simulink model "Wahadlo_model_lin"  (R2015a)
settings: Solver=ode45  SolverMode=SingleTasking  StartTime=0.0  StopTime=20  FixedStep=0.001  RelTol=1e-3  AbsTol=1e-6
values from neighbouring files (symbols this model uses):
  l0 = [0 0 0 0]    [model_prep_lqr.m]    (also in model_prep_swingup.m)
undefined symbols (not defined in the file or in its folder): a, b, g, l, M, m, s, w
settings Model: ExtModeTrigDuration=12000  ExtModeTrigLevel=0.400000  Creator=jims  LastModifiedBy=omicronns
settings DataIOCC: ExternalInput=[]  InitialState=[]  LimitDataPoints=off  MaxDataPoints=5000  SignalLoggingSaveFormat=ModelDataLogs  SaveOutput=off  SaveTime=off  SignalLoggingName=sigsOut
settings OptimizationCC: BooleanDataType=off  ExpressionDepthLimit=2147483647  InitFltsAndDblsToZero=on
settings DebuggingCC: SaveWithParameterizedLinksMsg=none  UnderspecifiedInitializationDetection=Classic  MergeDetectMultiDrivingBlocksExec=none  SignalResolutionControl=TryResolveAllWithWarning  MultiTaskDSMMsg=warning  MultiTaskCondExecSysMsg=none  IntegerOverflowMsg=none  FcnCallInpInsideContextMsg=UseLocalSettings  StateNameClashWarn=warning  IntegerSaturationMsg=none
settings HardwareCC: ProdBitPerLong=64  ProdBitPerPointer=64  ProdIntDivRoundTo=Zero  ProdEndianess=LittleEndian  ProdWordSize=64  ProdHWDeviceType=Intel->x86-64  TargetBitPerLong=64  TargetBitPerPointer=64  TargetIntDivRoundTo=Zero  TargetEndianess=LittleEndian  TargetWordSize=64  TargetHWDeviceType=Intel->x86-64
settings RTWCC: SystemTargetFile=rtwin.tlc  TemplateMakefile=RTDAC_win.tmf  Description=Real-Time Windows Target
settings RTWinTargetCC: TargetFcnLib=ansi_tfl_tmw.mat  TargetPreCompLibLocation=C:\Program Files\MATLAB\MATLAB Production Server\R2015a\toolbox\sldrt\lib\win64  ModelReferenceCompliant=off  CompOptLevelCompliant=off

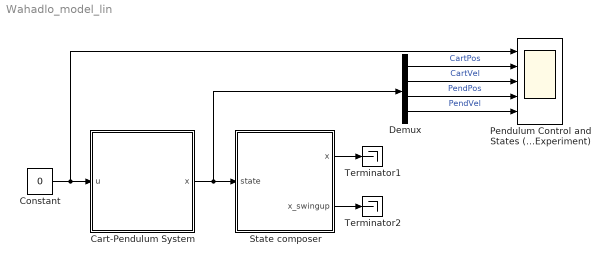
== system Wahadlo_model_lin ==
  Cart-Pendulum System : Subsystem
  Constant : Constant  Value=0
  Demux : Demux
  Pendulum Control and States (Experiment) : Scope  NumInputPorts=5
      settings: TimeRange=10  YMin=-0.2~-0.01~-0.04~0~-10  YMax=0.1~0.004999999999999999~0.02~6~10  SaveName=P1_Data  MaxDataPoints=50000
  State composer : Subsystem
  Terminator1 : Terminator
  Terminator2 : Terminator
  wires:
  Demux/4 -> Pendulum Control and States (Experiment)/5  "PendVel"
  Demux/3 -> Pendulum Control and States (Experiment)/4  "PendPos"
  Demux/2 -> Pendulum Control and States (Experiment)/3  "CartVel"
  Demux/1 -> Pendulum Control and States (Experiment)/2  "CartPos"
  Constant/1 -> Cart-Pendulum System/1(u), Pendulum Control and States (Experiment)/1
  Cart-Pendulum System/1(x) -> Demux/1, State composer/1(state)
  State composer/1(x) -> Terminator1/1
  State composer/2(x_swingup) -> Terminator2/1

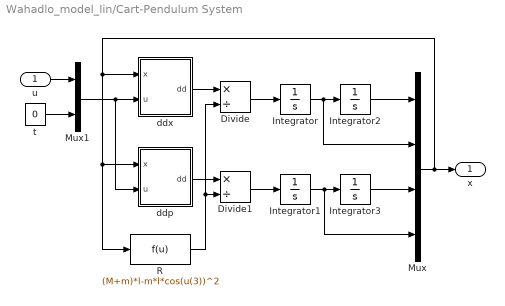
== system Wahadlo_model_lin/Cart-Pendulum System ==
  u : Inport
  Divide : Product  Inputs=*/
  Divide1 : Product  Inputs=*/
  Integrator : Integrator  InitialCondition=l0(2)
  Integrator1 : Integrator  InitialCondition=l0(4)
  Integrator2 : Integrator  InitialCondition=l0(1)
  Integrator3 : Integrator  InitialCondition=l0(3)
  Mux : Mux
  Mux1 : Mux  Inputs=2
  R : Fcn  Expr=(M+m)*l-m*l*cos(u(3))^2
  ddp : Subsystem
  ddx : Subsystem
  t : Constant  Value=0
  x : Outport
  wires:
  Integrator/1 -> Mux/2, Integrator2/1
  Integrator1/1 -> Mux/4, Integrator3/1
  Integrator2/1 -> Mux/1
  Integrator3/1 -> Mux/3
  Mux/1 -> R/1, ddp/1(x), ddx/1(x), x/1
  ddx/1(dd) -> Divide/1
  ddp/1(dd) -> Divide1/1
  Divide/1 -> Integrator/1
  Divide1/1 -> Integrator1/1
  R/1 -> Divide/2, Divide1/2
  Mux1/1 -> ddp/2(u), ddx/2(u)
  t/1 -> Mux1/2
  u/1 -> Mux1/1

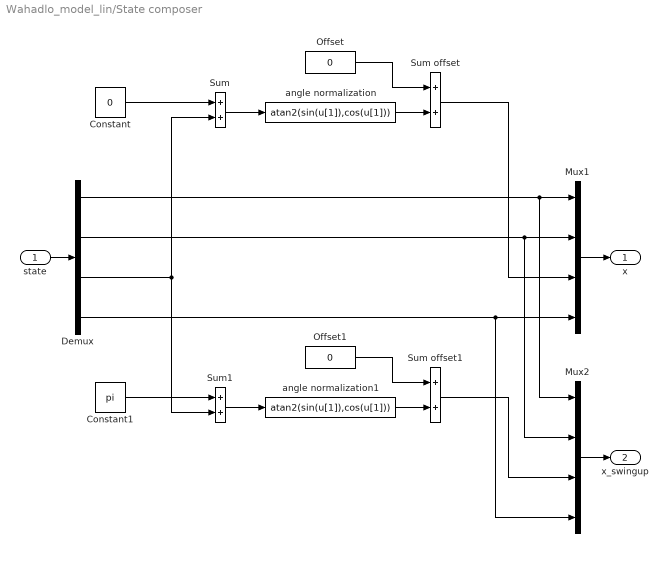
== system Wahadlo_model_lin/State composer ==
  state : Inport
  Constant : Constant  Value=0
  Constant1 : Constant  Value=pi
  Demux : Demux
  Mux1 : Mux
  Mux2 : Mux
  Offset : Constant  Value=0
  Offset1 : Constant  Value=0
  Sum : Sum  SaturateOnIntegerOverflow=on  InputSameDT=on  OutDataTypeStr=Inherit: Same as first input
  Sum offset : Sum  SaturateOnIntegerOverflow=on  InputSameDT=on  OutDataTypeStr=Inherit: Same as first input
  Sum offset1 : Sum  SaturateOnIntegerOverflow=on  InputSameDT=on  OutDataTypeStr=Inherit: Same as first input
  Sum1 : Sum  SaturateOnIntegerOverflow=on  InputSameDT=on  OutDataTypeStr=Inherit: Same as first input
  angle normalization : Fcn  Expr=atan2(sin(u[1]),cos(u[1]))
  angle normalization1 : Fcn  Expr=atan2(sin(u[1]),cos(u[1]))
  x : Outport  InitialOutput=0
  x_swingup : Outport  Port=2  InitialOutput=0
  wires:
  angle normalization/1 -> Sum offset/2
  Offset/1 -> Sum offset/1
  Sum/1 -> angle normalization/1
  Constant/1 -> Sum/1
  Mux1/1 -> x/1
  angle normalization1/1 -> Sum offset1/2
  Offset1/1 -> Sum offset1/1
  Sum1/1 -> angle normalization1/1
  Constant1/1 -> Sum1/1
  Mux2/1 -> x_swingup/1
  Sum offset/1 -> Mux1/3
  state/1 -> Demux/1
  Demux/3 -> Sum1/2, Sum/2
  Demux/2 -> Mux1/2, Mux2/2
  Demux/1 -> Mux1/1, Mux2/1
  Demux/4 -> Mux2/4, Mux1/4
  Sum offset1/1 -> Mux2/3

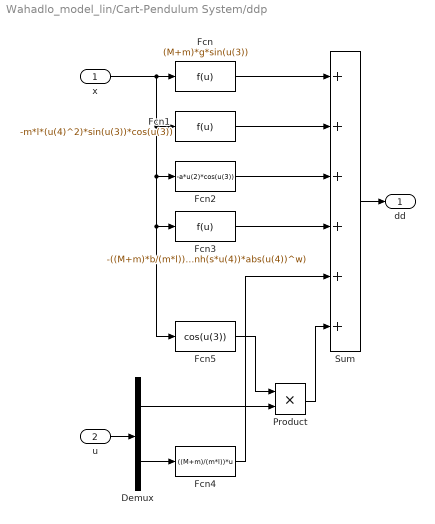
== system Wahadlo_model_lin/Cart-Pendulum System/ddp ==
  x : Inport
  u : Inport  Port=2
  Demux : Demux  Outputs=2
  Fcn : Fcn  Expr=(M+m)*g*sin(u(3))
  Fcn1 : Fcn  Expr=-m*l*(u(4)^2)*sin(u(3))*cos(u(3))
  Fcn2 : Fcn  Expr=-a*u(2)*cos(u(3))
  Fcn3 : Fcn  Expr=-((M+m)*b/(m*l))*(tanh(s*u(4))*abs(u(4))^w)
  Fcn4 : Fcn  Expr=((M+m)/(m*l))*u
  Fcn5 : Fcn  Expr=cos(u(3))
  Product : Product
  Sum : Sum  Inputs=++++++
  dd : Outport
  wires:
  u/1 -> Demux/1
  Fcn5/1 -> Product/1
  Fcn/1 -> Sum/1
  Fcn1/1 -> Sum/2
  Fcn2/1 -> Sum/3
  Fcn3/1 -> Sum/4
  x/1 -> Fcn3/1, Fcn5/1, Fcn2/1, Fcn1/1, Fcn/1
  Product/1 -> Sum/6
  Sum/1 -> dd/1
  Demux/2 -> Fcn4/1
  Demux/1 -> Product/2
  Fcn4/1 -> Sum/5

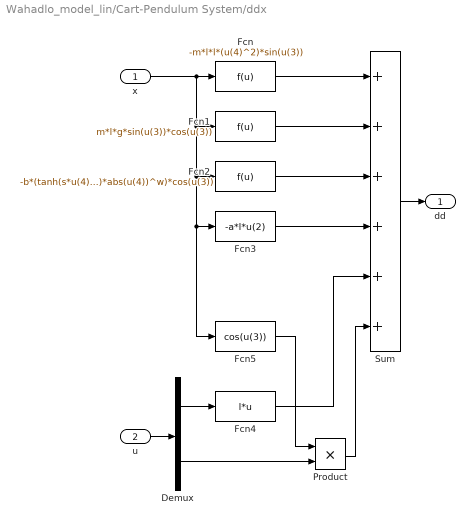
== system Wahadlo_model_lin/Cart-Pendulum System/ddx ==
  x : Inport
  u : Inport  Port=2
  Demux : Demux  Outputs=2
  Fcn : Fcn  Expr=-m*l*l*(u(4)^2)*sin(u(3))
  Fcn1 : Fcn  Expr=m*l*g*sin(u(3))*cos(u(3))
  Fcn2 : Fcn  Expr=-b*(tanh(s*u(4))*abs(u(4))^w)*cos(u(3))
  Fcn3 : Fcn  Expr=-a*l*u(2)
  Fcn4 : Fcn  Expr=l*u
  Fcn5 : Fcn  Expr=cos(u(3))
  Product : Product
  Sum : Sum  Inputs=++++++
  dd : Outport
  wires:
  u/1 -> Demux/1
  Demux/1 -> Fcn4/1
  Fcn5/1 -> Product/1
  Demux/2 -> Product/2
  Fcn/1 -> Sum/1
  Fcn1/1 -> Sum/2
  Fcn2/1 -> Sum/3
  Fcn3/1 -> Sum/4
  x/1 -> Fcn3/1, Fcn5/1, Fcn2/1, Fcn1/1, Fcn/1
  Fcn4/1 -> Sum/5
  Product/1 -> Sum/6
  Sum/1 -> dd/1
